simulink model "Torrico2019SimuEx3"  (R2018a)
settings: Solver=VariableStepAuto  StartTime=0.0  StopTime=Tsim  RelTol=1e-3
StopFcn:
  | plotSimu3
values from neighbouring files (symbols this model uses):
  distAmp = -0.06    [Torrico2019Example3.m]
  distTime = 20    [Torrico2019Example3.m]
  noiseTime = 55    [Torrico2019Example1.m]    (also in Torrico2019Example2.m = 99; Torrico2019Example3.m = 35)
  refAmp = 0.2    [Torrico2019Example3.m]
  Ts = 0.1    [Bismark2019.m]    (also in Torrico2019.m; Torrico2019Example1.m; Torrico2019Example2.m = 0.05; Torrico2019Example3.m = 0.01)
  uLim = 90.15    [Torrico2019Example3.m]
libraries: cstblocks x4, simulink x1
settings Model: Creator=aluno-2  LastModifiedBy=adriano

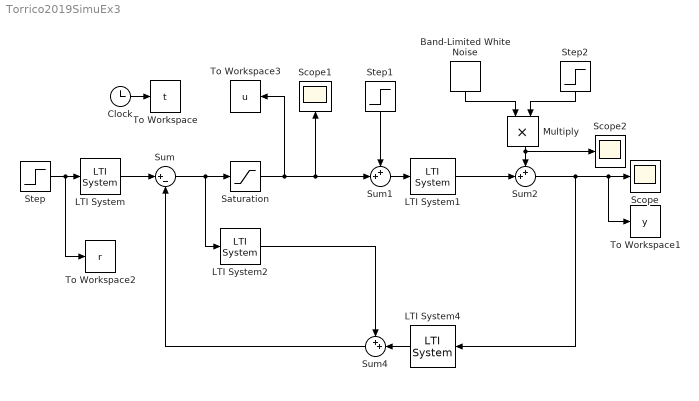
== system Torrico2019SimuEx3 ==
  Band-Limited White Noise : simulink/Sources/Band-Limited White Noise  Cov=noisePower  Ts=Ts  seed=[23341]
  Clock : Clock
  LTI System : cstblocks/LTI System  sys=F  IC=[]
  LTI System1 : cstblocks/LTI System  sys=P1z  IC=[]
  LTI System2 : cstblocks/LTI System  sys=S  IC=[]
  LTI System4 : cstblocks/LTI System  sys=V  IC=[]
  Multiply : Product
  Saturation : Saturate  UpperLimit=uLim  LowerLimit=-uLim
  Scope : Scope
  Scope1 : Scope
  Scope2 : Scope
  Step : Step  Time=0  After=refAmp  SampleTime=0
  Step1 : Step  Time=distTime  After=distAmp  SampleTime=0
  Step2 : Step  Time=noiseTime  SampleTime=0
  Sum : Sum  Inputs=|+-
  Sum1 : Sum  Inputs=++|
  Sum2 : Sum  Inputs=++|
  Sum4 : Sum  Inputs=++|
  To Workspace : ToWorkspace  VariableName=t  SampleTime=Ts
  To Workspace1 : ToWorkspace  VariableName=y  SampleTime=Ts
  To Workspace2 : ToWorkspace  VariableName=r  SampleTime=Ts
  To Workspace3 : ToWorkspace  VariableName=u  SampleTime=Ts
  wires:
  Step/1 -> To Workspace2/1, LTI System/1
  LTI System/1 -> Sum/1
  Sum1/1 -> LTI System1/1
  LTI System1/1 -> Sum2/2
  Sum4/1 -> Sum/2
  Sum2/1 -> LTI System4/1, To Workspace1/1, Scope/1
  LTI System2/1 -> Sum4/1
  LTI System4/1 -> Sum4/2
  Clock/1 -> To Workspace/1
  Sum/1 -> Saturation/1, LTI System2/1
  Band-Limited White Noise/1 -> Multiply/1
  Step2/1 -> Multiply/2
  Multiply/1 -> Scope2/1, Sum2/1
  Saturation/1 -> To Workspace3/1, Sum1/2, Scope1/1
  Step1/1 -> Sum1/1
